simulink model "untitled"  (R2021a)
settings: Solver=VariableStepAuto  StartTime=0.0  StopTime=10.0  RelTol=1e-3
undefined symbols (not defined in the file or in its folder): A, B
settings Model: Creator=VTX  LastModifiedBy=VTX

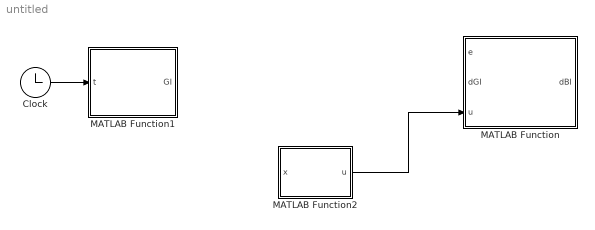
== system untitled ==
  Clock : Clock
  MATLAB Function : MATLAB Function  TreatAsAtomicUnit=on
  MATLAB Function1 : MATLAB Function  TreatAsAtomicUnit=on
  MATLAB Function2 : MATLAB Function  TreatAsAtomicUnit=on
  wires:
  Clock/1 -> MATLAB Function1/1(t)
  MATLAB Function2/1(u) -> MATLAB Function/3(u)

== matlab function untitled/MATLAB Function2 ==
  data: x input; u output; K parameter
function u = fcn(x,K)
    u = K*x;
end

== matlab function untitled/MATLAB Function ==
  data: e input; dBI output; dGI input; u input; A parameter; B parameter
function dBI = fcn(e,dGI,u,A, B)
    dBI = dGI - (A*e + B*u);
end

== matlab function untitled/MATLAB Function1 ==
  data: t input; GI output
function GI = fcn(t)
    GI = [sin(0.5*t) cos(0.25*t) 5*sin(0.25*t) (sin(t)+sin(0.5*t)) 2*cos(t) cos(t)]';
end
